simulink library "ilcUpdate_cl"  (R2018b)
settings: Solver=VariableStepAuto  StartTime=0.0  StopTime=10.0  RelTol=1e-3
undefined symbols (not defined in the file): forgFact, Ts
libraries: ilcUpdateLaw_cl x1, rlsGradientEst_cl x1
settings Model: Creator=mcobb  LastModifiedBy=mcobb

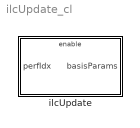
== system ilcUpdate_cl ==
  ilcUpdate : Subsystem  mask{initBasisParams=0, lrn=0, AdaptationParameter=forgFact, trstRgn=0, wtNoise=0, Ts=Ts}
      mask prompts: initBasisParams "Init Basis Params"; lrn "Gradient Based Learning Gain"; AdaptationParameter "Controllib:blocks:recursiveEstimationMaskAdaptationParameterFF"; trstRgn "Trust Region Dimensions"; wtNoise "White Noise Dimensions"; Ts "Sample Time"
      mask TypeOptions lrn: ilcUpdateLaw/lrn
      mask TypeOptions AdaptationParameter: rlsGradientEst/AdaptationParameter
      mask TypeOptions trstRgn: ilcUpdateLaw/trstRgn
      mask TypeOptions wtNoise: ilcUpdateLaw/wtNoise
      mask TypeOptions Ts: rlsGradientEst/Ts
      mask DialogControl AdaptationParameter Prompt: Forgetting Factor:

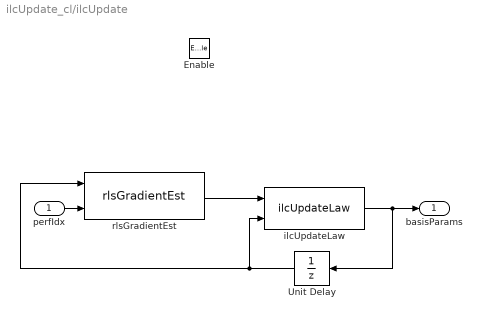
== system ilcUpdate_cl/ilcUpdate ==
  perfIdx : Inport
  Enable : EnablePort
  Unit Delay : UnitDelay  InitialCondition=initBasisParams  SampleTime=-1
  ilcUpdateLaw : ilcUpdateLaw_cl/ilcUpdateLaw  lrn=lrn  trstRgn=trstRgn  wtNoise=wtNoise
  rlsGradientEst : rlsGradientEst_cl/rlsGradientEst  InitialParameterData=initBasisParams  AdaptationParameter=AdaptationParameter  Ts=Ts
  basisParams : Outport  InitialOutput=initBasisParams
  wires:
  rlsGradientEst/1 -> ilcUpdateLaw/1
  perfIdx/1 -> rlsGradientEst/2
  ilcUpdateLaw/1 -> Unit Delay/1, basisParams/1
  Unit Delay/1 -> rlsGradientEst/1, ilcUpdateLaw/2
